simulink model "ask"  (R2023b)
settings: Solver=VariableStepAuto  StartTime=0.0  StopTime=10.0  RelTol=1e-3
settings Model: Creator=ASUS  LastModifiedBy=ASUS

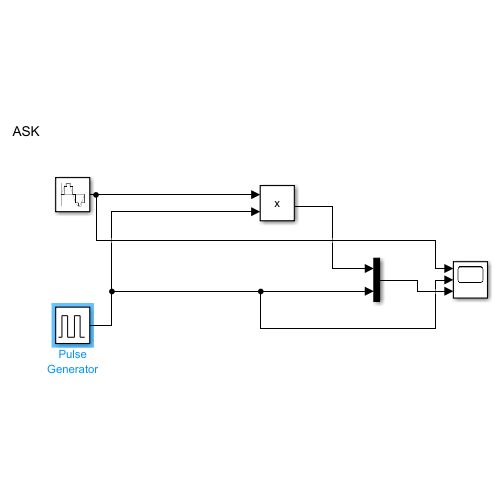
[thumbnail: Simulink's stored preview of the top-level diagram]
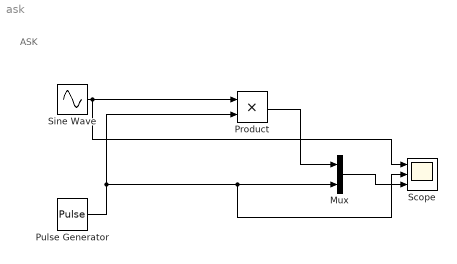
== system ask ==
  note: ASK
  Mux : Mux  Inputs=2
  Product : Product
  Pulse Generator : DiscretePulseGenerator  PulseType=Time based  PulseWidth=50
  Scope : Scope  NumInputPorts=3
  Sine Wave : Sin  Frequency=50  SampleTime=0.01
  wires:
  Mux/1 -> Scope/3
  Product/1 -> Mux/1
  Sine Wave/1 -> Scope/1, Product/1
  Pulse Generator/1 -> Scope/2, Mux/2, Product/2
